simulink model "Final_model"  (R2023a)
settings: Solver=FixedStepAuto  StartTime=0.0  StopTime=10.0  RelTol=1e-3
undefined symbols (not defined in the file): Acceleration, Distance_from_Home, Has_fallen, Inclination, Is_overspeeding, Off_Alarm, Switch, Transmit_data, untitled, Velocity
libraries: androiduilib x8, androidcommunicationlib x4, androidsensorlib x3, androidaudiovideolib x3, simulink x2
settings Model: Creator=Abhishek  LastModifiedBy=Abhishek
settings OptimizationCC: EnhancedBackFolding=on  PassReuseOutputArgsAs=Individual arguments  ZeroExternalMemoryAtStartup=off  ZeroInternalMemoryAtStartup=off  MaxStackSize=64  OptimizeBlockOrder=speed  DifferentSizesBufferReuse=on  OptimizationCustomize=off  EfficientTunableParamExpr=on
settings DebuggingCC: ParameterTunabilityLossMsg=error
settings HardwareCC: ProdBitPerPointer=32  ProdBitPerSizeT=32  ProdBitPerPtrDiffT=32  ProdLargestAtomicInteger=Long  ProdLargestAtomicFloat=Double  ProdWordSize=32  ProdHWDeviceType=ARM Compatible->ARM Cortex  UseEmbeddedCoderFeatures=off  UseSimulinkCoderFeatures=off
settings SFSimCC: MATLABDynamicMemAlloc=off
settings RTWCC: Description=Embedded Coder  SystemTargetFile=ert.tlc  HardwareBoard=Android Device  TLCOptions="-aInlineSetEventsForThisBaseRateFcn=TLC_FALSE -aSuppressMultiTaskScheduler=TLC_FALSE  -aRateBasedStepFcn=0"  TemplateMakefile=ert_default_tmf  RTWVerbose=off  Toolchain=Android SDK/NDK Tools
settings CodeAppCC: ForceParamTrailComments=on  IgnoreCustomStorageClasses=off  OperatorAnnotations=on  SimulinkDataObjDesc=on  SFDataObjDesc=on  InsertBlockDesc=on
settings ERTTargetCC: SupportNonInlinedSFcns=on

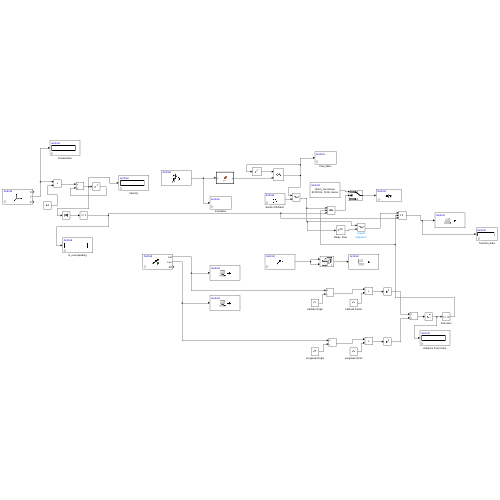
[thumbnail: Simulink's stored preview of the top-level diagram]
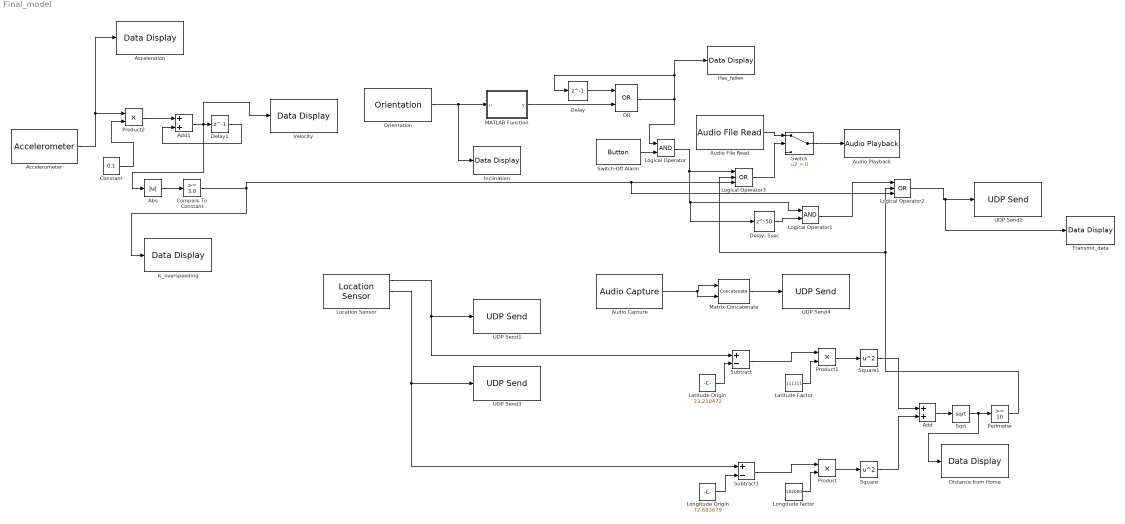
== system Final_model ==
  Abs : Abs  SaturateOnIntegerOverflow=off
  Acceleration : androiduilib/Data Display  DataDisplayId=untitled/Acceleration  Format=Float  Precision=6  SimulateUsing=Code generation  blockPlatform=Android
  Accelerometer : androidsensorlib/Accelerometer  OutputVector=off  SampleTime=0.1  BlockPlatform=Android
  Add : Sum
  Add1 : Sum
  Audio Capture : androidaudiovideolib/Audio Capture  SampleFreq=24000  FrameSize=2400  SampleTime=0.1  SimulateUsing=Code generation  DeviceStr=0  QueueDuration=0  BlockPlatform=Android  AudioSamplingFreq=44100
  Audio File Read : androidaudiovideolib/Audio File Read  FileName=C:\Users\Abhishek\Music\Alarm_sound.wav  FrameSize=4100
  Audio Playback : androidaudiovideolib/Audio Playback  SampleFreq=44100  AudioSamplingFreq=44100  SampleTime=0.1  DeviceStr=0  QueueDuration=0  BlockPlatform=Android
  Compare To Constant : simulink/Logic and Bit Operations/Compare To Constant  relop=>=  const=3.0  OutDataTypeStr=boolean
  Constant : Constant  Value=0.1
  Delay : Delay  DelayLength=1  InitialCondition=0
  Delay1 : Delay  DelayLength=1  InitialCondition=0
  Delay: 5sec : Delay  DelayLength=50  InitialCondition=0
  Distance from Home : androiduilib/Data Display  DataDisplayId=untitled/Distance_from_Home  Format=Float  Precision=6  SimulateUsing=Code generation  blockPlatform=Android
  Has_fallen : androiduilib/Data Display  DataDisplayId=untitled/Has_fallen  Format=Float  Precision=6  SimulateUsing=Code generation  blockPlatform=Android
  Inclination : androiduilib/Data Display  DataDisplayId=untitled/Inclination  Format=Float  Precision=6  SimulateUsing=Code generation  blockPlatform=Android
  Is_overspeeding : androiduilib/Data Display  DataDisplayId=untitled/Is_overspeeding  Format=Float  Precision=6  SimulateUsing=Code generation  blockPlatform=Android
  Latitude Factor : Constant  Value=111111
  Latitude Origin : Constant  Value=23.210472
  Location Sensor : androidsensorlib/Location Sensor  OutputVector=off  SampleTime=0.1  BlockPlatform=Android
  Logical Operator : Logic  AllPortsSameDT=off  OutDataTypeStr=boolean
  Logical Operator1 : Logic  AllPortsSameDT=off  OutDataTypeStr=boolean
  Logical Operator2 : Logic  Operator=OR  Inputs=3  AllPortsSameDT=off  OutDataTypeStr=boolean
  Logical Operator3 : Logic  Operator=OR  Inputs=3  AllPortsSameDT=off  OutDataTypeStr=boolean
  Longitude Origin : Constant  Value=72.683679
  Longitude factor : Constant  Value=102000
  MATLAB Function : MATLAB Function  TreatAsAtomicUnit=on
  Matrix Concatenate : Concatenate  Mode=Multidimensional array
  OR : Logic  Operator=OR  AllPortsSameDT=off  OutDataTypeStr=boolean
  Orientation : androidsensorlib/Orientation  SampleTime=0.1
  Perimeter : simulink/Logic and Bit Operations/Compare To Constant  relop=>=  const=10  OutDataTypeStr=boolean
  Product : Product
  Product1 : Product
  Product2 : Product
  Sqrt : Sqrt
  Square : Math  Operator=square
  Square1 : Math  Operator=square
  Subtract : Sum  Inputs=+-
  Subtract1 : Sum  Inputs=+-
  Switch : Switch  Criteria=u2 > Threshold  SaturateOnIntegerOverflow=off  InputSameDT=off
  Switch-Off Alarm : androiduilib/Button  ButtonState=Pressed  ButtonId=untitled/Switch-Off_Alarm  State=on  SampleTime=0.1  BlockPlatform=Android
  Transmit_data : androiduilib/Data Display  DataDisplayId=untitled/Transmit_data  Format=Float  Precision=6  SimulateUsing=Code generation  blockPlatform=Android
  UDP Send1 : androidcommunicationlib/UDP Send  remoteURL='10.7.14.46'  remotePort=30001  localURL='0.0.0.0'  localPortSource=Automatically determine  localPort=-1  sampletime=-1  blockPlatform=Android  separateLengthPort=0
  UDP Send2 : androidcommunicationlib/UDP Send  remoteURL='10.7.14.46'  remotePort=30012  localURL='0.0.0.0'  localPortSource=Automatically determine  localPort=-1  sampletime=-1  blockPlatform=Android  separateLengthPort=0
  UDP Send3 : androidcommunicationlib/UDP Send  remoteURL='10.7.14.46'  remotePort=30002  localURL='0.0.0.0'  localPortSource=Automatically determine  localPort=-1  sampletime=-1  blockPlatform=Android  separateLengthPort=0
  UDP Send4 : androidcommunicationlib/UDP Send  remoteURL='10.7.14.46'  remotePort=30011  localURL='0.0.0.0'  localPortSource=Automatically determine  localPort=-1  sampletime=-1  blockPlatform=Android  separateLengthPort=0
  Velocity : androiduilib/Data Display  DataDisplayId=untitled/Velocity  Format=Float  Precision=6  SimulateUsing=Code generation  blockPlatform=Android
  wires:
  MATLAB Function/1(y) -> OR/2
  Location Sensor/2 -> Subtract1/1, UDP Send3/1
  Square1/1 -> Add/1
  Longitude Origin/1 -> Subtract1/2
  Orientation/1 -> Inclination/1, MATLAB Function/1(u)
  Sqrt/1 -> Distance from Home/1, Perimeter/1
  Add/1 -> Sqrt/1
  Latitude Origin/1 -> Subtract/2
  Logical Operator1/1 -> Logical Operator2/1
  Subtract/1 -> Product1/1
  Delay/1 -> OR/1
  Logical Operator/1 -> Delay: 5sec/1, Logical Operator1/1, Logical Operator3/1
  Latitude Factor/1 -> Product1/2
  Square/1 -> Add/2
  Audio Capture/1 -> Matrix Concatenate/2, Matrix Concatenate/1
  Switch/1 -> Audio Playback/1
  Location Sensor/1 -> Subtract/1, UDP Send1/1
  Delay: 5sec/1 -> Logical Operator1/2
  Subtract1/1 -> Product/1
  Switch-Off Alarm/1 -> Logical Operator/2
  Logical Operator2/1 -> Transmit_data/1, UDP Send2/1
  Perimeter/1 -> Logical Operator3/2, Logical Operator2/2
  Product1/1 -> Square1/1
  Matrix Concatenate/1 -> UDP Send4/1
  Audio File Read/1 -> Switch/1
  Logical Operator3/1 -> Switch/2
  OR/1 -> Delay/1, Has_fallen/1, Logical Operator/1
  Product/1 -> Square/1
  Longitude factor/1 -> Product/2
  Abs/1 -> Compare To Constant/1
  Add1/1 -> Abs/1, Velocity/1, Delay1/1
  Product2/1 -> Add1/1
  Compare To Constant/1 -> Is_overspeeding/1, Logical Operator2/3, Logical Operator3/3
  Accelerometer/2 -> Product2/1, Acceleration/1
  Delay1/1 -> Add1/2
  Constant/1 -> Product2/2

== matlab function Final_model/MATLAB Function ==
  data: u input; y output
function y = fcn(u)

inc = u(2);
if inc<-65 || inc> 65
    y = 1;
else
    y = 0;
end
